simulink model "VPD_lab_4_linear"  (R2022b)
settings: Solver=VariableStepAuto  StartTime=0.0  StopTime=50  RelTol=1e-3
undefined symbols (not defined in the file): B, goal_x, goal_y, J, K_r, K_s, ke, km, L, r, R
settings Model: Creator=Alex  LastModifiedBy=Alex

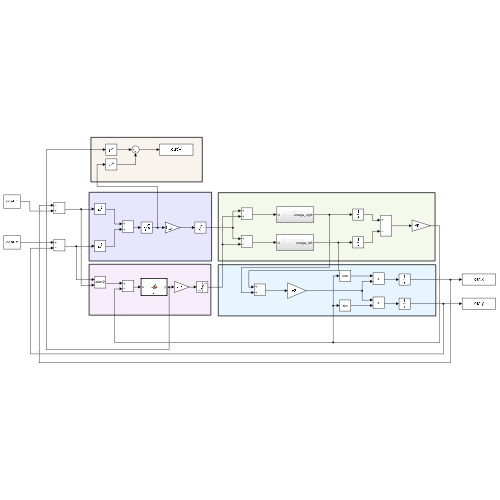
[thumbnail: Simulink's stored preview of the top-level diagram]
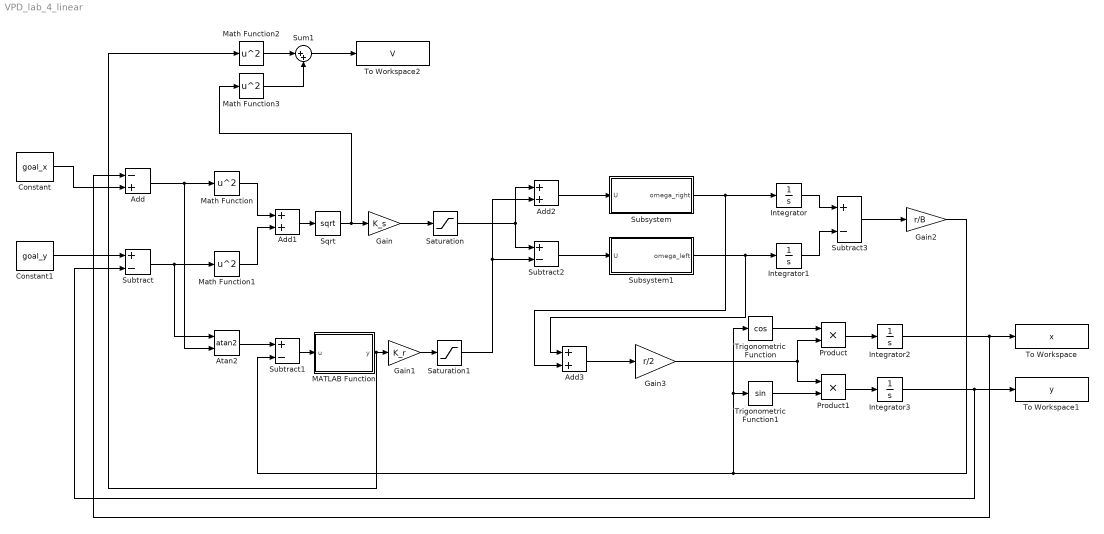
== system VPD_lab_4_linear ==
  Add : Sum  Inputs=-+
  Add1 : Sum
  Add2 : Sum
  Add3 : Sum
  Atan2 : Trigonometry  Operator=atan2
  Constant : Constant  Value=goal_x
  Constant1 : Constant  Value=goal_y
  Gain : Gain  Gain=K_s
  Gain1 : Gain  Gain=K_r
  Gain2 : Gain  Gain=r/B
  Gain3 : Gain  Gain=r/2
  Integrator{,1..3} (4 alike) : Integrator
  MATLAB Function : MATLAB Function  TreatAsAtomicUnit=on
  Math Function{,1..3} (4 alike) : Math  Operator=square
  Product : Product
  Product1 : Product
  Saturation : Saturate  UpperLimit=6.4  LowerLimit=-6.4
  Saturation1 : Saturate  UpperLimit=1.6  LowerLimit=-1.6
  Sqrt : Sqrt
  Subsystem : Subsystem
  Subsystem1 : Subsystem
  Subtract{,1..3} (4 alike) : Sum  Inputs=+-
  Sum1 : Sum  Inputs=|++
  To Workspace : ToWorkspace  VariableName=x  SaveFormat=Timeseries  SampleTime=-1
  To Workspace1 : ToWorkspace  VariableName=y  SaveFormat=Timeseries  SampleTime=-1
  To Workspace2 : ToWorkspace  VariableName=V  SaveFormat=Timeseries  SampleTime=-1
  Trigonometric Function : Trigonometry  Operator=cos
  Trigonometric Function1 : Trigonometry
  wires:
  Add/1 -> Atan2/2, Math Function/1
  Subtract/1 -> Math Function1/1, Atan2/1
  Constant/1 -> Add/2
  Constant1/1 -> Subtract/1
  Math Function1/1 -> Add1/2
  Math Function/1 -> Add1/1
  Add1/1 -> Sqrt/1
  Sqrt/1 -> Math Function3/1, Gain/1
  Gain/1 -> Saturation/1
  Atan2/1 -> Subtract1/1
  Subtract1/1 -> MATLAB Function/1(u)
  MATLAB Function/1(y) -> Math Function2/1, Gain1/1
  Gain1/1 -> Saturation1/1
  Saturation/1 -> Add2/1, Subtract2/1
  Saturation1/1 -> Subtract2/2, Add2/2
  Integrator/1 -> Subtract3/1
  Integrator1/1 -> Subtract3/2
  Subtract3/1 -> Gain2/1
  Trigonometric Function/1 -> Product/1
  Trigonometric Function1/1 -> Product1/2
  Gain3/1 -> Product1/1, Product/2
  Product/1 -> Integrator2/1
  Product1/1 -> Integrator3/1
  Gain2/1 -> Subtract1/2, Trigonometric Function1/1, Trigonometric Function/1
  Add3/1 -> Gain3/1
  Subsystem/1(omega_right) -> Integrator/1, Add3/2
  Add2/1 -> Subsystem/1(U)
  Subtract2/1 -> Subsystem1/1(U)
  Subsystem1/1(omega_left) -> Add3/1, Integrator1/1
  Integrator2/1 -> Add/1, To Workspace/1
  Integrator3/1 -> Subtract/2, To Workspace1/1
  Math Function2/1 -> Sum1/1
  Math Function3/1 -> Sum1/2
  Sum1/1 -> To Workspace2/1

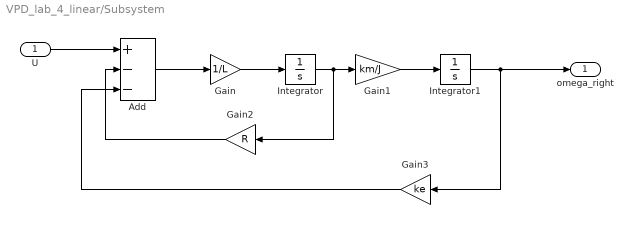
== system VPD_lab_4_linear/Subsystem ==
  U : Inport
  Add : Sum  Inputs=+--
  Gain : Gain  Gain=1/L
  Gain1 : Gain  Gain=km/J
  Gain2 : Gain  Gain=R
  Gain3 : Gain  Gain=ke
  Integrator : Integrator
  Integrator1 : Integrator
  omega_right : Outport
  wires:
  Gain/1 -> Integrator/1
  Integrator1/1 -> Gain3/1, omega_right/1
  Add/1 -> Gain/1
  Gain2/1 -> Add/2
  Integrator/1 -> Gain2/1, Gain1/1
  Gain1/1 -> Integrator1/1
  Gain3/1 -> Add/3
  U/1 -> Add/1

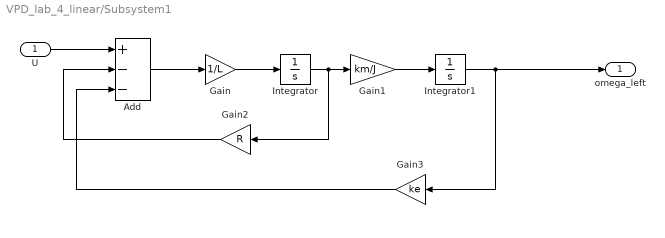
== system VPD_lab_4_linear/Subsystem1 ==
  U : Inport
  Add : Sum  Inputs=+--
  Gain : Gain  Gain=1/L
  Gain1 : Gain  Gain=km/J
  Gain2 : Gain  Gain=R
  Gain3 : Gain  Gain=ke
  Integrator : Integrator
  Integrator1 : Integrator
  omega_left : Outport
  wires:
  U/1 -> Add/1
  Add/1 -> Gain/1
  Gain/1 -> Integrator/1
  Integrator/1 -> Gain2/1, Gain1/1
  Gain2/1 -> Add/2
  Gain1/1 -> Integrator1/1
  Integrator1/1 -> omega_left/1, Gain3/1
  Gain3/1 -> Add/3

== matlab function VPD_lab_4_linear/MATLAB Function ==
  data: u input; y output
function y = fcn(u)
if (u <=-pi)
    y=u+2*pi;
elseif (u>=pi)
    y=u-2*pi;
else
    y=u;
end
